simulink model "AAI_VVI_Mode"  (R2023b)
settings: Solver=FixedStepAuto  StartTime=0.0  StopTime=10.0  FixedStep=1e-3  RelTol=1e-3  EnableMultiTasking=on
undefined symbols (not defined in the file): D0, D1, D11, D12, D13, D2, D3, D6, D8, D9, PTA0, PTA1, PTB9, PTC16, PTC17, PTC2, PTC4, PTD1, PTD2, PTD3
libraries: frdmk64flib x10
settings Model: ExtModeTrigDuration=5  Creator=stivb  LastModifiedBy=stivb
settings OptimizationCC: EnhancedBackFolding=on  PassReuseOutputArgsAs=Individual arguments  ZeroExternalMemoryAtStartup=off  ZeroInternalMemoryAtStartup=off  MaxStackSize=64  OptimizeBlockOrder=speed  DifferentSizesBufferReuse=on  OptimizationCustomize=off  EfficientTunableParamExpr=on
settings DebuggingCC: ParameterTunabilityLossMsg=error
settings HardwareCC: ProdBitPerPointer=32  ProdBitPerSizeT=32  ProdBitPerPtrDiffT=32  ProdLargestAtomicInteger=Long  ProdLargestAtomicFloat=Double  ProdWordSize=32  ProdHWDeviceType=ARM Compatible->ARM Cortex
settings SFSimCC: MATLABDynamicMemAlloc=off
settings RTWCC: Description=Embedded Coder  SystemTargetFile=ert.tlc  HardwareBoard=NXP FRDM-K64F  TLCOptions="-aInlineSetEventsForThisBaseRateFcn=TLC_FALSE -aSuppressMultiTaskScheduler=TLC_FALSE  -aRateBasedStepFcn=0"  TemplateMakefile=ert_default_tmf  Toolchain=GNU Tools for ARM Embedded Processors
settings CodeAppCC: ForceParamTrailComments=on  IgnoreCustomStorageClasses=off  OperatorAnnotations=on  SimulinkDataObjDesc=on  SFDataObjDesc=on  InsertBlockDesc=on
settings ERTTargetCC: ExtModeTransport=4  ExtModeMexFile=sendToCommService

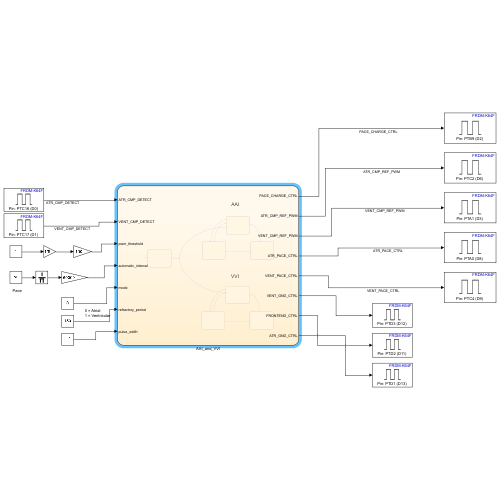
[thumbnail: Simulink's stored preview of the top-level diagram]
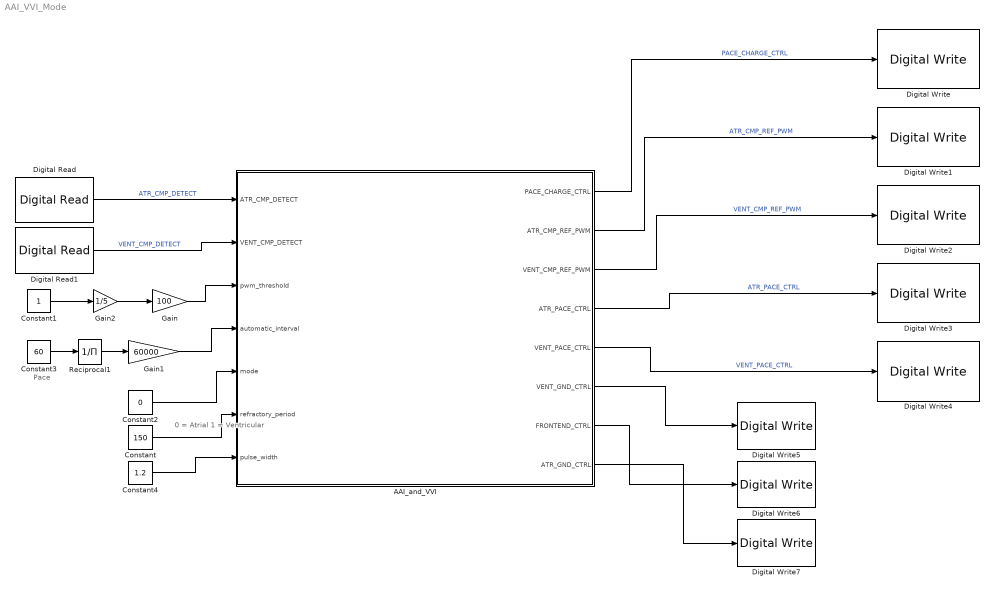
== system AAI_VVI_Mode ==
  note: Pace
  note: 0 = Atrial
      | 1 = Ventricular
  AAI_and_VVI : Stateflow chart  TreatAsAtomicUnit=on
  Constant : Constant  Value=150
  Constant1 : Constant
  Constant2 : Constant  Value=0
  Constant3 : Constant  Value=60
  Constant4 : Constant  Value=1.2
  Digital Read : frdmk64flib/Digital Read  Whichpin=PTC16 (D0)  SampleTime=-1
  Digital Read1 : frdmk64flib/Digital Read  Whichpin=PTC17 (D1)  SampleTime=-1
  Digital Write : frdmk64flib/Digital Write  Whichpin=PTB9 (D2)
  Digital Write1 : frdmk64flib/Digital Write  Whichpin=PTC2 (D6)
  Digital Write2 : frdmk64flib/Digital Write  Whichpin=PTA1 (D3)
  Digital Write3 : frdmk64flib/Digital Write  Whichpin=PTA0 (D8)
  Digital Write4 : frdmk64flib/Digital Write  Whichpin=PTC4 (D9)
  Digital Write5 : frdmk64flib/Digital Write  Whichpin=PTD3 (D12)
  Digital Write6 : frdmk64flib/Digital Write  Whichpin=PTD2 (D11)
  Digital Write7 : frdmk64flib/Digital Write  Whichpin=PTD1 (D13)
  Gain : Gain  Gain=100
  Gain1 : Gain  Gain=60000
  Gain2 : Gain  Gain=1/5
  Reciprocal1 : Product  Inputs=/
  wires:
  AAI_and_VVI/1(PACE_CHARGE_CTRL) -> Digital Write/1  "PACE_CHARGE_CTRL"
  AAI_and_VVI/2(ATR_CMP_REF_PWM) -> Digital Write1/1  "ATR_CMP_REF_PWM"
  AAI_and_VVI/3(VENT_CMP_REF_PWM) -> Digital Write2/1  "VENT_CMP_REF_PWM"
  AAI_and_VVI/4(ATR_PACE_CTRL) -> Digital Write3/1  "ATR_PACE_CTRL"
  AAI_and_VVI/5(VENT_PACE_CTRL) -> Digital Write4/1  "VENT_PACE_CTRL"
  Constant2/1 -> AAI_and_VVI/5(mode)
  Gain1/1 -> AAI_and_VVI/4(automatic_interval)
  Reciprocal1/1 -> Gain1/1
  Gain2/1 -> Gain/1
  Gain/1 -> AAI_and_VVI/3(pwm_threshold)
  Constant/1 -> AAI_and_VVI/6(refractory_period)
  Digital Read1/1 -> AAI_and_VVI/2(VENT_CMP_DETECT)  "VENT_CMP_DETECT"
  Digital Read/1 -> AAI_and_VVI/1(ATR_CMP_DETECT)  "ATR_CMP_DETECT"
  Constant1/1 -> Gain2/1
  Constant3/1 -> Reciprocal1/1
  Constant4/1 -> AAI_and_VVI/7(pulse_width)
  AAI_and_VVI/6(VENT_GND_CTRL) -> Digital Write5/1
  AAI_and_VVI/7(FRONTEND_CTRL) -> Digital Write6/1
  AAI_and_VVI/8(ATR_GND_CTRL) -> Digital Write7/1

== stateflow chart AAI_VVI_Mode/AAI_and_VVI ==
  note: AAI
  note: Safe start entry; since hysteresis pacing allows for waiting a period of time longer than the refractory period, we are okay with waiting a refractory period of time before we start pacing. This also ensures that the capacitors are appropriately charged to allow for proper pacing.
  state Refractory_and_charging
    entry:
    FRONTEND_CTRL = 0;
    %Charge C22
    ATR_PACE_CTRL = 0;
    PACE_CHARGE_CTRL = 1;
    %Discharge C21
    ATR_GND_CTRL= 1;
    % Setup sensing pins
    ATR_CMP_REF_PWM = pwm_threshold;
  note: Detected a pace, so go back to refractory state to wait
      | the appropriate refractory time interval
  state Sensing
    entry:
    FRONTEND_CTRL = 1;
  state Pacing
    entry:
    PACE_CHARGE_CTRL = 0;
    ATR_PACE_CTRL = 1;
    ATR_GND_CTRL = 0;
  state Mode_select_state_entry_point
  note: VVI
  note: Safe start entry; since hysteresis pacing allows for waiting a period of time longer than the refractory period, we are okay with waiting a refractory period of time before we start pacing. This also ensures that the capacitors are appropriately charged to allow for proper pacing.
  state Refractory_and_charging1
    entry:
    FRONTEND_CTRL = 0;
    %Charge C22
    VENT_PACE_CTRL = 0;
    PACE_CHARGE_CTRL = 1;
    %Discharge C21
    VENT_GND_CTRL= 1;
    % Setup sensing pins
    VENT_CMP_REF_PWM = pwm_threshold;
  note: Detected a pace, so go back to refractory state to wait
      | the appropriate refractory time interval
  state Sensing1
    entry:
    FRONTEND_CTRL = 1;
  state Pacing1
    entry:
    PACE_CHARGE_CTRL = 0;
    VENT_PACE_CTRL = 1;
    VENT_GND_CTRL = 0;
  Refractory_and_charging -> Sensing : after(refractory_period, msec)
  Sensing -> Refractory_and_charging [order 1] : [ATR_CMP_DETECT == true]
  Pacing -> Refractory_and_charging : after(pulse_width, msec)
  (junction 36) -> Refractory_and_charging [order 1] : [mode == 0]
  Sensing -> Pacing [order 2] : after(automatic_interval - refractory_period - pulse_width, msec)
  (default) -> Mode_select_state_entry_point
  Mode_select_state_entry_point -> (junction 36)
  (junction 36) -> Refractory_and_charging1 [order 2] : [mode == 1]
  Refractory_and_charging1 -> Sensing1 : after(refractory_period, msec)
  Sensing1 -> Refractory_and_charging1 [order 1] : [VENT_CMP_DETECT == true]
  Pacing1 -> Refractory_and_charging1 : after(pulse_width, msec)
  Sensing1 -> Pacing1 [order 2] : after(automatic_interval - refractory_period - pulse_width, msec)
  data: ATR_CMP_DETECT input; VENT_CMP_DETECT input; PACE_CHARGE_CTRL output; ATR_CMP_REF_PWM output; VENT_CMP_REF_PWM output; ATR_PACE_CTRL output; VENT_PACE_CTRL output; pwm_threshold input; automatic_interval input; mode input; refractory_period input; VENT_GND_CTRL output; FRONTEND_CTRL output; ATR_GND_CTRL output; pulse_width input
